simulink model "vbyfcontrolim_trials"  (R2016a)
settings: Solver=ode4  StartTime=0.0  StopTime=20  FixedStep=Ts  RelTol=1e-3
values from neighbouring files (symbols this model uses):
  Cdc = 100e-6    (= 0.0001)    [control_simulation_parameters.m]    (also in pmsm_vbyf_sim_parameters.m = 1.5e-05; vbyfcontrolim_sim.m)
  deltad = delta*180/pi    [control_simulation_parameters.m]    (also in pmsm_vbyf_sim_parameters.m)
  Ef = 155    [control_simulation_parameters.m]    (also in pmsm_vbyf_sim_parameters.m = 80)
  fout = 50    [control_simulation_parameters.m]    (also in pmsm_vbyf_sim_parameters.m = 100; vbyfcontrolim_sim.m)
  frated = 50    [vbyfcontrolim_sim.m]
  Ls = 13.8e-3    (= 0.0138)    [control_simulation_parameters.m]
  ma = Vt*sqrt(3)/(Vdcm*0.612)    [control_simulation_parameters.m]    (also in pmsm_vbyf_sim_parameters.m; vbyfcontrolim_sim.m = 0.9)
  phase = [0 90 0 90]    [control_simulation_parameters.m]    (also in pmsm_vbyf_sim_parameters.m = [0])
  Rin = 10    [control_simulation_parameters.m]    (also in pmsm_vbyf_sim_parameters.m = 1; vbyfcontrolim_sim.m = 1e-06)
  Ripth = 0.08    [control_simulation_parameters.m]    (also in pmsm_vbyf_sim_parameters.m; vbyfcontrolim_sim.m)
  Rs = 1e-3    (= 0.001)    [control_simulation_parameters.m]
  Tload = 30    [pmsm_vbyf_sim_parameters.m]    (also in vbyfcontrolim_sim.m = 10)
  Ts = 100e-9    (= 1e-07)    [control_simulation_parameters.m]    (also in pmsm_vbyf_sim_parameters.m = 1e-06; vbyfcontrolim_sim.m = 1e-06)
  VbyfFreqSteps = 2    [vbyfcontrolim_sim.m]
  VbyfStepTime = 0.2    [vbyfcontrolim_sim.m]
  Vdc = 300    [control_simulation_parameters.m]    (also in pmsm_vbyf_sim_parameters.m = 270; vbyfcontrolim_sim.m = 750)
  Vin = Vdc + Rin*(Pout/Vdc)    (= 366.666666667)    [control_simulation_parameters.m]    (also in pmsm_vbyf_sim_parameters.m = 276.981317008; vbyfcontrolim_sim.m = 750)
  wout = 2*pi*fout    (= 314.159265359)    [control_simulation_parameters.m]    (also in pmsm_vbyf_sim_parameters.m = 628.318530718; vbyfcontrolim_sim.m)
undefined symbols (not defined in the file or in its folder): Lload, Rload
libraries: powerlib x25, powerlib_meascontrol x13, simulink x4, dspsigops x4
settings Model: SimulationMode=accelerator  Creator=ugurm  LastModifiedBy=admin
settings DataIOCC: LimitDataPoints=on  SaveFormat=Array
settings DebuggingCC: UnderspecifiedInitializationDetection=Classic  MergeDetectMultiDrivingBlocksExec=none  SolverPrmCheckMsg=warning  StateNameClashWarn=warning
settings HardwareCC: ProdBitPerPointer=32  ProdLargestAtomicFloat=None  ProdIntDivRoundTo=Undefined  ProdEndianess=Unspecified  ProdWordSize=32  ProdHWDeviceType=32-bit Generic
settings ModelReferenceCC: PropagateSignalLabelsOutOfModel=off
settings SimscapeCC: SimscapeNormalizeSystem=off

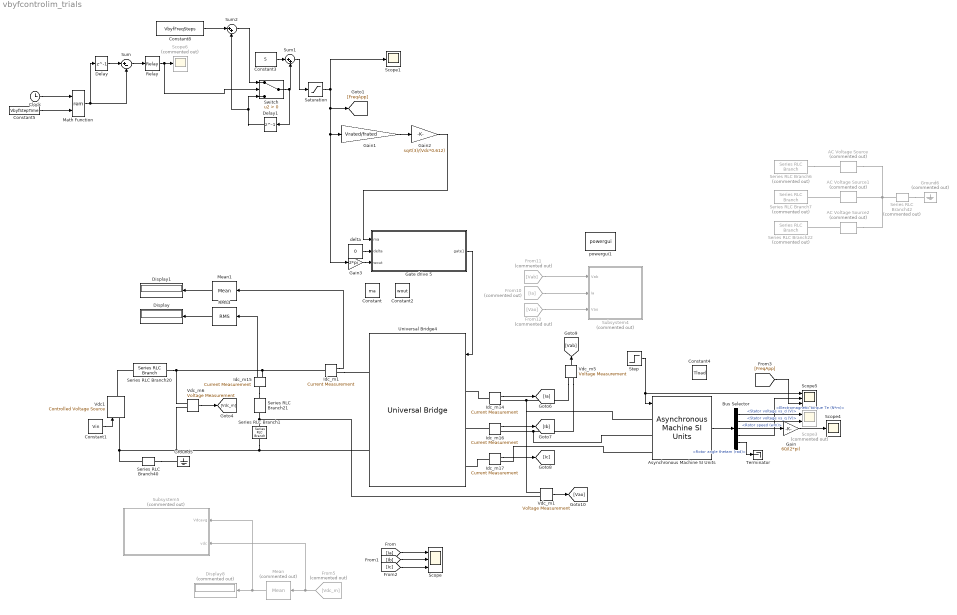
== system vbyfcontrolim_trials ==
  AC Voltage Source : powerlib/Electrical Sources/AC Voltage Source  Commented=on  Amplitude=Ef*sqrt(2)  Phase=0  Frequency=fout  SampleTime=0  Measurements=None  BusType=swing  Pref=10e3  Qref=0  Qmin=-inf  Qmax=+inf
  AC Voltage Source1 : powerlib/Electrical Sources/AC Voltage Source  Commented=on  Amplitude=Ef*sqrt(2)  Phase=-120  Frequency=fout  SampleTime=0  Measurements=None  BusType=swing  Pref=10e3  Qref=0  Qmin=-inf  Qmax=+inf
  AC Voltage Source2 : powerlib/Electrical Sources/AC Voltage Source  Commented=on  Amplitude=Ef*sqrt(2)  Phase=-240  Frequency=fout  SampleTime=0  Measurements=None  BusType=swing  Pref=10e3  Qref=0  Qmin=-inf  Qmax=+inf
  Asynchronous Machine SI Units : powerlib/Machines/Asynchronous Machine SI Units  RotorType=Squirrel-cage  PresetModel=No  MechanicalLoad=Torque Tm  ShowDetailedParameters=on  ReferenceFrame=Synchronous  Units=SI  MeasurementBus=off  NominalParameters=[4000 400 50]  Stator=[1.405 0.005839]  Rotor=[1.395 0.005839]  Cage1=[0.4155 0.002066]  Cage2=[0.4168 0.0003495]  Lm=0.1722  Mechanical=[0.0131 0.002985 2]  PolePairs=2  InitialConditions=[0 0 0 0 0 0 0 0]  SimulateSaturation=off  Saturation=[14.03593122, 27.81365428, 53.79336849, 72.68890987, 97.98006896, 148.6815601, 215.7428561, 302.9841135, 428.7778367 ; 230, 322, 414, 460, 506, 552, 598, 644, 690]  LoadFlowParameters=1492000  TsPowergui=0  TsBlock=-1  IterativeModel=Trapezoidal non iterative  IterativeDiscreteModel=Trapezoidal non iterative  Pmec=1.492e+006
  Bus Selector : BusSelector  OutputSignals=Stator measurements.Stator voltage vs_d (V),Stator measurements.Stator voltage vs_q (V),Mechanical.Rotor speed (wm),Mechanical.Electromagnetic torque Te (N*m),Mechanical.Rotor angle thetam (rad)
  Clock : Clock
  Constant : Constant  Value=ma
  Constant1 : Constant  Value=Vin
  Constant2 : Constant  Value=wout
  Constant3 : Constant  Value=5
  Constant4 : Constant  Value=Tload
  Constant5 : Constant  Value=VbyfStepTime
  Constant8 : Constant  Value=VbyfFreqSteps
  Delay : Delay  DelayLength=1
  Delay1 : Delay  DelayLength=1
  Display : Display
  Display1 : Display
  Display8 : Display  Commented=on
  From10 : From  Commented=on  GotoTag=Ia
  From11 : From  Commented=on  GotoTag=Vab
  From12 : From  Commented=on  GotoTag=Vao
  From5 : From  Commented=on  GotoTag=Vdc_m
  Gain : Gain  Gain=60/(2*pi)
  Gain1 : Gain  Gain=Vrated/frated
  Gain2 : Gain  Gain=sqrt(3)/(Vdc*0.612)
  Gain3 : Gain  Gain=2*pi
  Gate drive 5 : Subsystem
  Ground5 : powerlib/Elements/Ground  LConnTagsString=a
  Ground6 : powerlib/Elements/Ground  Commented=on  LConnTagsString=a
  Idc_m{1,14..17} (5 alike) : powerlib/Measurements/Current Measurement  PhasorSimulation=off  OutputType=Complex  PSBequivalent=0
  Math Function : Math  Operator=rem  SaturateOnIntegerOverflow=on
  Mean : powerlib_meascontrol/Measurements/Mean  Commented=on  Freq=fout  Vinit=0  Ts=0
  Mean1 : powerlib_meascontrol/Measurements/Mean  Freq=fout  Vinit=0  Ts=0
  RMS3 : powerlib_meascontrol/Measurements/RMS  TrueRMS=on  Freq=fout  RMSInit=0  Ts=0
  Relay : Relay
  Saturation : Saturate  UpperLimit=frated  LowerLimit=0
  Scope : Scope  NumInputPorts=3
  Scope1 : Scope
  Scope3 : Scope  Commented=on  NumInputPorts=2
  Scope4 : Scope
  Scope5 : Scope  NumInputPorts=3
  Scope6 : Scope  Commented=on
  Series RLC Branch1 : powerlib/Elements/Series RLC Branch  LConnTagsString=__new0  RConnTagsString=__new0  BranchType=C  Resistance=Rload  Inductance=Lload  SetiL0=off  InitialCurrent=0  Capacitance=Cdc*2  Setx0=off  InitialVoltage=0  Measurements=None
  Series RLC Branch20 : powerlib/Elements/Series RLC Branch  LConnTagsString=__new0  RConnTagsString=__new0  BranchType=R  Resistance=Rin  Inductance=Lload  SetiL0=off  InitialCurrent=0  Capacitance=1e-6  Setx0=off  InitialVoltage=0  Measurements=None
  Series RLC Branch21 : powerlib/Elements/Series RLC Branch  LConnTagsString=__new0  RConnTagsString=__new0  BranchType=C  Resistance=Rload  Inductance=Lload  SetiL0=off  InitialCurrent=0  Capacitance=Cdc*2  Setx0=off  InitialVoltage=0  Measurements=None
  Series RLC Branch22 : powerlib/Elements/Series RLC Branch  Commented=on  LConnTagsString=__new0  RConnTagsString=__new0  BranchType=RL  Resistance=Rs  Inductance=Ls  SetiL0=off  InitialCurrent=0  Capacitance=1e-6  Setx0=off  InitialVoltage=0  Measurements=None
  Series RLC Branch40 : powerlib/Elements/Series RLC Branch  LConnTagsString=__new0  RConnTagsString=__new0  BranchType=R  Resistance=1e12  Inductance=Lload  SetiL0=off  InitialCurrent=0  Capacitance=1e-6  Setx0=off  InitialVoltage=0  Measurements=None
  Series RLC Branch42 : powerlib/Elements/Series RLC Branch  Commented=on  LConnTagsString=__new0  RConnTagsString=__new0  BranchType=R  Resistance=1e12  Inductance=Lload  SetiL0=off  InitialCurrent=0  Capacitance=1e-6  Setx0=off  InitialVoltage=0  Measurements=None
  Series RLC Branch6 : powerlib/Elements/Series RLC Branch  Commented=on  LConnTagsString=__new0  RConnTagsString=__new0  BranchType=RL  Resistance=Rs  Inductance=Ls  SetiL0=off  InitialCurrent=0  Capacitance=1e-6  Setx0=off  InitialVoltage=0  Measurements=None
  Series RLC Branch7 : powerlib/Elements/Series RLC Branch  Commented=on  LConnTagsString=__new0  RConnTagsString=__new0  BranchType=RL  Resistance=Rs  Inductance=Ls  SetiL0=off  InitialCurrent=0  Capacitance=1e-6  Setx0=off  InitialVoltage=0  Measurements=None
  Step : Step  Time=2  After=Tload  SampleTime=0
  Subsystem4 : Subsystem  Commented=on
  Subsystem5 : Subsystem  Commented=on
  Sum : Sum  Inputs=|+-
  Sum1 : Sum  Inputs=|++
  Sum2 : Sum  Inputs=|++
  Switch : Switch  Criteria=u2 > Threshold
  Terminator : Terminator
  Universal Bridge4 : powerlib/Power Electronics/Universal Bridge  Arms=3  SnubberResistance=1e5  SnubberCapacitance=inf  Device=IGBT / Diodes  Ron=1e-6  Lon=0  ForwardVoltages="[  0  0  ]"  ForwardVoltage=0  GTOparameters=[ 10e-6 , 20e-6 ]  IGBTparameters=[0,0]  Measurements=None  Measurements_2=None  converterType=Rectifier
  Vdc1 : powerlib/Electrical Sources/Controlled Voltage Source  Initialize=off  Source_Type=DC  Amplitude=200  Phase=0  Frequency=0  Measurements=None
  Vdc_m1 : powerlib/Measurements/Voltage Measurement  PhasorSimulation=off  OutputType=Complex  PSBequivalent=0
  Vdc_m5 : powerlib/Measurements/Voltage Measurement  PhasorSimulation=off  OutputType=Complex  PSBequivalent=0
  Vdc_m6 : powerlib/Measurements/Voltage Measurement  PhasorSimulation=off  OutputType=Complex  PSBequivalent=0
  delta : Constant  Value=0
  powergui1 : powerlib/powergui  Priority=1  SimulationMode=Discrete  SampleTime=Ts  frequency=60  Iterations=50  frequencyindice=0  Pbase=100e6  ErrMax=1e-4  UnitsV=kV  UnitsW=MW  buscounter=0  FunctionMessages=off  echomessages=off  EnableUseOfTLC=off  CurrentSourceSwitches=off  DisableSnubberDevices=off  DisableRonSwitches=off  DisableVfSwitches=off  DisplayEquations=off  AutomaticDiscreteSolvers=off  SolverType=Tustin  Interpol=off  ExternalGateDelay=off  methode=off  Ts=0  x0status=blocks  SPID=off  SwTol=0  HookPort=off  NonlinearTolerance=0  nMaxIteration=15  ContinueOnMaxIteration=off  RestoreLinks=warning  ResistiveCurrentMeasurement=off  Frange=[0:2:500]  Ylog=off  Xlog=on  ShowGrid=off  save=off  variable=ZData  structure=Vdc  ZoomFFT=off  StartTime=0.04  cycles=5  DisplayStyle=5  fundamental=50  FreqAxis=off  MaxFrequency=30000  frequencyindicesteady=1  RmsSteady=1  display=off
  wires:
  Gate drive 5/1(gate1) -> Universal Bridge4/1
  Constant1/1 -> Vdc1/1
  Idc_m15/1 -> RMS3/1
  Vdc_m6/1 -> [Vdc_m]
  RMS3/1 -> Display/1
  Mean/1 -> Subsystem5/1(Vdcavg), Display8/1
  Idc_m1/1 -> Mean1/1
  Mean1/1 -> Display1/1
  Idc_m14/1 -> [Ia]
  From5/1 -> Subsystem5/2(vdc), Mean/1
  From10/1 -> Subsystem4/2(Ia)
  Idc_m16/1 -> [Ib]
  Idc_m17/1 -> [Ic]
  From11/1 -> Subsystem4/1(Vab)
  From12/1 -> Subsystem4/3(Vao)
  Vdc_m5/1 -> [Vab]
  Vdc_m1/1 -> [Vao]
  [Ia] -> Scope/1
  [Ic] -> Scope/3
  [Ib] -> Scope/2
  delta/1 -> Gate drive 5/2(delta)
  Asynchronous Machine SI Units/1 -> Bus Selector/1
  Bus Selector/1 -> Scope3/1  "<Stator voltage vs_d (V)>"
  Bus Selector/2 -> Scope3/2  "<Stator voltage vs_q (V)>"
  Bus Selector/3 -> Gain/1  "<Rotor speed (wm)>"
  Bus Selector/4 -> Scope5/2  "<Electromagnetic torque Te (N*m)>"
  Bus Selector/5 -> Terminator/1  "<Rotor angle thetam (rad)>"
  Gain/1 -> Scope4/1
  Clock/1 -> Math Function/1
  Constant5/1 -> Math Function/2
  Math Function/1 -> Sum/2, Delay/1
  Delay/1 -> Sum/1
  Sum/1 -> Relay/1
  Relay/1 -> Switch/2, Scope6/1
  Sum2/1 -> Switch/1
  Constant8/1 -> Sum2/1
  Delay1/1 -> Switch/3, Sum2/2
  Switch/1 -> Sum1/2, Delay1/1
  Gain1/1 -> Gain2/1
  Gain2/1 -> Gate drive 5/1(ma)
  Gain3/1 -> Gate drive 5/3(wout)
  Saturation/1 -> [FreqApp], Gain3/1, Gain1/1, Scope1/1
  Step/1 -> Scope5/1, Asynchronous Machine SI Units/1
  [FreqApp] -> Scope5/3
  Constant3/1 -> Sum1/1
  Sum1/1 -> Saturation/1
  connections:
  Vdc_m5/LConn1 -- Asynchronous Machine SI Units/LConn1 -- Vdc_m1/LConn1 -- Idc_m14/RConn1
  Universal Bridge4/RConn2 -- Vdc_m6/LConn2 -- Vdc1/LConn1 -- Series RLC Branch40/LConn1 -- Series RLC Branch1/RConn1
  Series RLC Branch42/RConn1 -- Ground6/LConn1
  Series RLC Branch40/RConn1 -- Ground5/LConn1
  Idc_m14/LConn1 -- Universal Bridge4/LConn1
  Idc_m15/LConn1 -- Series RLC Branch21/LConn1
  Vdc1/RConn1 -- Series RLC Branch20/LConn1
  Series RLC Branch6/RConn1 -- AC Voltage Source/RConn1
  AC Voltage Source1/RConn1 -- Series RLC Branch7/RConn1
  AC Voltage Source2/RConn1 -- Series RLC Branch22/RConn1
  Series RLC Branch42/LConn1 -- AC Voltage Source/LConn1 -- AC Voltage Source2/LConn1 -- AC Voltage Source1/LConn1
  Idc_m16/LConn1 -- Universal Bridge4/LConn2
  Idc_m17/LConn1 -- Universal Bridge4/LConn3
  Vdc_m5/LConn2 -- Asynchronous Machine SI Units/LConn2 -- Idc_m16/RConn1
  Idc_m1/RConn1 -- Universal Bridge4/RConn1
  Idc_m1/LConn1 -- Series RLC Branch20/RConn1 -- Vdc_m6/LConn1 -- Idc_m15/RConn1
  Series RLC Branch1/LConn1 -- Vdc_m1/LConn2 -- Series RLC Branch21/RConn1
  Asynchronous Machine SI Units/LConn3 -- Idc_m17/RConn1

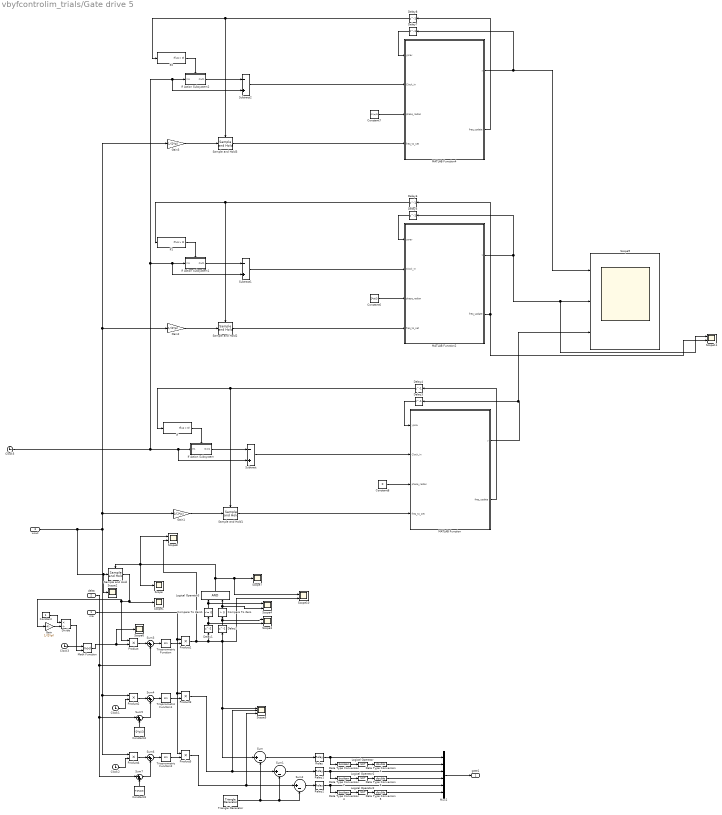
== system vbyfcontrolim_trials/Gate drive 5 ==
  ma : Inport
  delta : Inport  Port=2
  wout : Inport  Port=3
  Clock{1..3,5} (4 alike) : Clock
  Compare To Zero : simulink/Logic and Bit Operations/Compare To Zero  relop=>  OutDataTypeStr=boolean
  Compare To Zero1 : simulink/Logic and Bit Operations/Compare To Zero  relop=<=  OutDataTypeStr=boolean
  Constant : Constant
  Constant3 : Constant  Value=+2*pi/3
  Constant4 : Constant  Value=-2*pi/3
  Constant6 : Constant  Value=2*pi/3
  Constant7 : Constant  Value=-2*pi/3
  Constant8 : Constant  Value=0
  Data Type Conversion : DataTypeConversion  OutDataTypeStr=boolean
  Data Type Conversion1 : DataTypeConversion  OutDataTypeStr=double
  Data Type Conversion2 : DataTypeConversion  OutDataTypeStr=boolean
  Data Type Conversion3 : DataTypeConversion  OutDataTypeStr=double
  Data Type Conversion4 : DataTypeConversion  OutDataTypeStr=boolean
  Data Type Conversion5 : DataTypeConversion  OutDataTypeStr=double
  Delay1 : Delay
  Delay{2..8} (7 alike) : Delay  DelayLength=1
  Divide : Product  Inputs=*/
  Gain{,1..3} (4 alike) : Gain  Gain=1/(2*pi)
  If : If  ShowElse=off
  If Action Subsystem : Subsystem  TreatAsAtomicUnit=on
  If Action Subsystem1 : Subsystem  TreatAsAtomicUnit=on
  If Action Subsystem2 : Subsystem  TreatAsAtomicUnit=on
  If1 : If  ShowElse=off
  If2 : If  ShowElse=off
  Logical Operator : Logic  Operator=NOT  AllPortsSameDT=off  OutDataTypeStr=boolean
  Logical Operator1 : Logic  Operator=NOT  AllPortsSameDT=off  OutDataTypeStr=boolean
  Logical Operator2 : Logic  Operator=NOT  AllPortsSameDT=off  OutDataTypeStr=boolean
  Logical Operator3 : Logic  AllPortsSameDT=off  OutDataTypeStr=boolean
  MATLAB Function : MATLAB Function  TreatAsAtomicUnit=on
  MATLAB Function2 : MATLAB Function  TreatAsAtomicUnit=on
  MATLAB Function4 : MATLAB Function  TreatAsAtomicUnit=on
  Math Function : Math  Operator=mod  SaturateOnIntegerOverflow=on
  Mux2 : Mux  Inputs=6
  Product{,1..5} (6 alike) : Product
  Relay : Relay
  Relay1 : Relay
  Relay2 : Relay
  Sample and Hold{,1..3} (4 alike) : dspsigops/Sample and Hold  trig=Rising edge  initCond=5*2*pi  latchinput=off
  Scope{,1..2,6..7} (5 alike) : Scope
  Scope{3..4,8,10..11} (5 alike) : Scope  NumInputPorts=2
  Scope5 : Scope  NumInputPorts=3
  Scope9 : Scope  NumInputPorts=3
  Subtract : Sum  Inputs=-+
  Subtract1 : Sum  Inputs=-+
  Subtract2 : Sum  Inputs=-+
  Sum : Sum  Inputs=|+-
  Sum1 : Sum  Inputs=|+-
  Sum2 : Sum  Inputs=|+-
  Sum{3..7} (5 alike) : Sum  Inputs=|++
  Triangle Generator : powerlib_meascontrol/Pulse & Signal Generators/Triangle Generator  Freq=fsw  Phase=phase(1)  Ts=Ts
  Trigonometric Function : Trigonometry
  Trigonometric Function1 : Trigonometry
  Trigonometric Function2 : Trigonometry
  gate1 : Outport
  wires:
  Triangle Generator/1 -> Sum1/2, Sum2/2, Sum/2
  Product3/1 -> Scope5/2, Sum1/1
  Product5/1 -> Scope5/3, Sum2/1
  Sum/1 -> Relay/1
  Sum1/1 -> Relay1/1
  Sum2/1 -> Relay2/1
  Data Type Conversion/1 -> Logical Operator/1
  Relay/1 -> Data Type Conversion/1, Mux2/1
  Logical Operator/1 -> Data Type Conversion1/1
  Data Type Conversion1/1 -> Mux2/2
  Data Type Conversion2/1 -> Logical Operator1/1
  Relay1/1 -> Data Type Conversion2/1, Mux2/3
  Logical Operator1/1 -> Data Type Conversion3/1
  Data Type Conversion3/1 -> Mux2/4
  Data Type Conversion4/1 -> Logical Operator2/1
  Relay2/1 -> Data Type Conversion4/1, Mux2/5
  Logical Operator2/1 -> Data Type Conversion5/1
  Data Type Conversion5/1 -> Mux2/6
  Mux2/1 -> gate1/1
  Trigonometric Function/1 -> Product1/2
  Sum3/1 -> Trigonometric Function/1
  Product/1 -> Sum3/1
  Clock1/1 -> Product2/2
  Trigonometric Function1/1 -> Product3/2
  Sum4/1 -> Trigonometric Function1/1
  Product2/1 -> Sum4/1
  Sum5/1 -> Sum4/2
  Constant4/1 -> Sum5/2
  ma/1 -> Product1/1, Product5/1, Product3/1
  delta/1 -> Sum7/1, Sum5/1, Sum3/2
  Clock2/1 -> Product4/2
  Trigonometric Function2/1 -> Product5/2
  Sum6/1 -> Trigonometric Function2/1
  Product4/1 -> Sum6/1
  Sum7/1 -> Sum6/2
  Constant3/1 -> Sum7/2
  Sample and Hold/1 -> Scope1/1, Product/1, Gain/1
  Product1/1 -> Scope8/2, Delay1/1, Scope10/2, Scope5/1, Sum/1, Delay2/1
  Delay1/1 -> Compare To Zero1/1, Scope3/2
  Compare To Zero/1 -> Scope4/2, Logical Operator3/2
  Compare To Zero1/1 -> Scope4/1, Logical Operator3/1
  Delay2/1 -> Scope3/1, Compare To Zero/1
  Gain/1 -> Divide/2
  Constant/1 -> Divide/1
  Divide/1 -> Math Function/2
  Clock3/1 -> Math Function/1
  Math Function/1 -> Scope6/1, Product/2
  Logical Operator3/1 -> Scope10/1, Scope7/1, Scope8/1, Scope/1, Sample and Hold/Trigger
  MATLAB Function/1(y) -> Scope9/3, Delay3/1
  Delay3/1 -> MATLAB Function/1(yprev)
  MATLAB Function/2(freq_update) -> Delay4/1
  Gain1/1 -> Sample and Hold1/1
  Sample and Hold1/1 -> MATLAB Function/4(freq_to_set)
  Delay4/1 -> Sample and Hold1/Trigger, If/1
  If Action Subsystem/1(Out1) -> Subtract/1
  If/1 -> If Action Subsystem/Action
  Subtract/1 -> MATLAB Function/2(Clock_In)
  Subtract1/1 -> MATLAB Function2/2(Clock_In)
  If1/1 -> If Action Subsystem1/Action
  If Action Subsystem1/1(Out1) -> Subtract1/1
  Delay6/1 -> If1/1, Sample and Hold2/Trigger
  Sample and Hold2/1 -> MATLAB Function2/4(freq_to_set)
  Gain2/1 -> Sample and Hold2/1
  MATLAB Function2/2(freq_update) -> Scope11/2, Delay6/1
  Delay5/1 -> MATLAB Function2/1(yprev)
  MATLAB Function2/1(y) -> Scope11/1, Scope9/2, Delay5/1
  MATLAB Function4/1(y) -> Scope9/1, Delay7/1
  Delay7/1 -> MATLAB Function4/1(yprev)
  MATLAB Function4/2(freq_update) -> Delay8/1
  If Action Subsystem2/1(Out1) -> Subtract2/1
  Sample and Hold3/1 -> MATLAB Function4/4(freq_to_set)
  Gain3/1 -> Sample and Hold3/1
  Delay8/1 -> If2/1, Sample and Hold3/Trigger
  Subtract2/1 -> MATLAB Function4/2(Clock_In)
  Clock5/1 -> Subtract/2, If Action Subsystem/1(In1), If Action Subsystem1/1(In1), Subtract1/2, If Action Subsystem2/1(In1), Subtract2/2
  If2/1 -> If Action Subsystem2/Action
  wout/1 -> Scope2/1, Sample and Hold/1, Product4/1, Product2/1, Gain3/1, Gain2/1, Gain1/1
  Constant6/1 -> MATLAB Function2/3(phase_radian)
  Constant7/1 -> MATLAB Function4/3(phase_radian)
  Constant8/1 -> MATLAB Function/3(phase_radian)

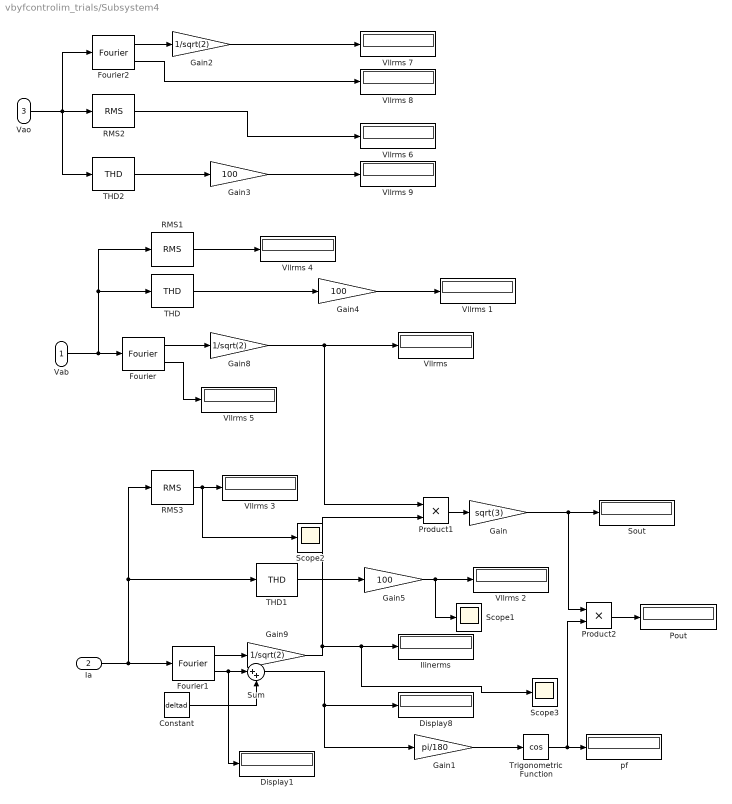
== system vbyfcontrolim_trials/Subsystem4 ==
  Vab : Inport
  Ia : Inport  Port=2
  Vao : Inport  Port=3
  Constant : Constant  Value=deltad
  Display1 : Display
  Display8 : Display
  Fourier : powerlib_meascontrol/Measurements/Fourier  Freq=fout  n=1  InInit=[0, 0]  Ts=Ts
  Fourier1 : powerlib_meascontrol/Measurements/Fourier  Freq=fout  n=1  InInit=[0, 0]  Ts=Ts
  Fourier2 : powerlib_meascontrol/Measurements/Fourier  Freq=fout  n=1  InInit=[0, 0]  Ts=Ts
  Gain : Gain  Gain=sqrt(3)
  Gain1 : Gain  Gain=pi/180
  Gain2 : Gain  Gain=1/sqrt(2)
  Gain3 : Gain  Gain=100
  Gain4 : Gain  Gain=100
  Gain5 : Gain  Gain=100
  Gain8 : Gain  Gain=1/sqrt(2)
  Gain9 : Gain  Gain=1/sqrt(2)
  "Ilinerms " : Display
  Pout : Display
  Product1 : Product
  Product2 : Product
  RMS1 : powerlib_meascontrol/Measurements/RMS  TrueRMS=on  Freq=fout  RMSInit=0  Ts=0
  RMS2 : powerlib_meascontrol/Measurements/RMS  TrueRMS=on  Freq=fout  RMSInit=0  Ts=0
  RMS3 : powerlib_meascontrol/Measurements/RMS  TrueRMS=on  Freq=fout  RMSInit=0  Ts=0
  Scope1 : Scope
  Scope2 : Scope
  Scope3 : Scope
  Sout : Display
      settings: Format=short_e
  Sum : Sum  Inputs=|++
  THD : powerlib_meascontrol/Measurements/THD  Freq=fout  Ts=0
  THD1 : powerlib_meascontrol/Measurements/THD  Freq=fout  Ts=0
  THD2 : powerlib_meascontrol/Measurements/THD  Freq=fout  Ts=0
  Trigonometric Function : Trigonometry  Operator=cos
  Vllrms {,1..9} (10 alike) : Display
  pf : Display
  wires:
  Gain8/1 -> Product1/1, "Vllrms "/1
  Gain9/1 -> Scope3/1, "Ilinerms "/1, Product1/2
  Ia/1 -> RMS3/1, THD1/1, Fourier1/1
  Fourier1/1 -> Gain9/1
  Vab/1 -> RMS1/1, THD/1, Fourier/1
  Fourier/1 -> Gain8/1
  Product1/1 -> Gain/1
  Gain/1 -> Product2/1, Sout/1
  Sum/1 -> Gain1/1, Display8/1
  Trigonometric Function/1 -> Product2/2, pf/1
  Gain1/1 -> Trigonometric Function/1
  Product2/1 -> Pout/1
  Fourier/2 -> Vllrms 5/1
  THD/1 -> Gain4/1
  THD1/1 -> Gain5/1
  Constant/1 -> Sum/2
  RMS3/1 -> Scope2/1, Vllrms 3/1
  RMS1/1 -> Vllrms 4/1
  Fourier1/2 -> Display1/1, Sum/1
  Vao/1 -> THD2/1, Fourier2/1, RMS2/1
  RMS2/1 -> Vllrms 6/1
  Fourier2/1 -> Gain2/1
  Fourier2/2 -> Vllrms 8/1
  Gain2/1 -> Vllrms 7/1
  THD2/1 -> Gain3/1
  Gain3/1 -> Vllrms 9/1
  Gain4/1 -> Vllrms 1/1
  Gain5/1 -> Scope1/1, Vllrms 2/1

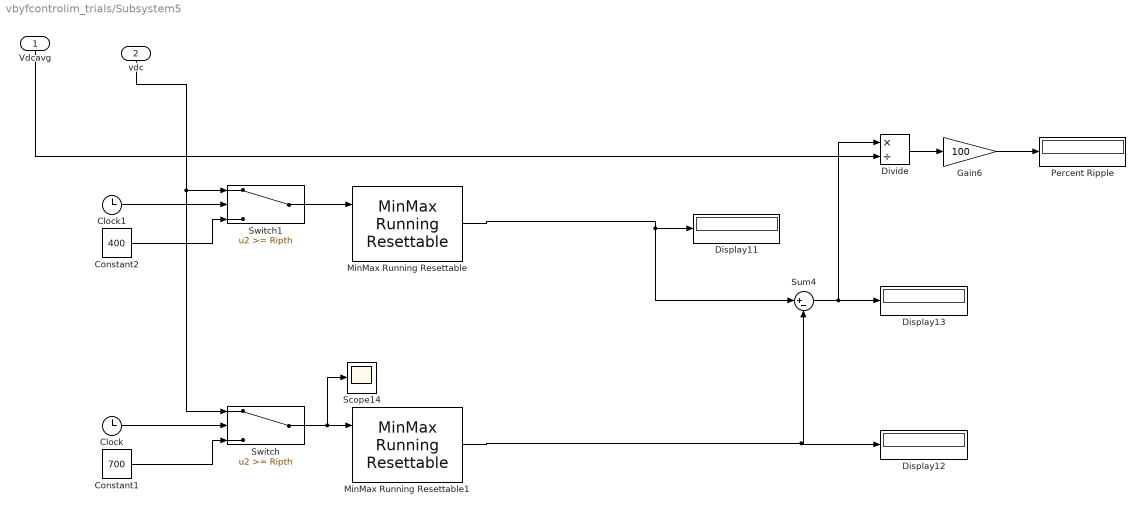
== system vbyfcontrolim_trials/Subsystem5 ==
  Vdcavg : Inport
  vdc : Inport  Port=2
  Clock : Clock
  Clock1 : Clock
  Constant1 : Constant  Value=700  SampleTime=Ts
  Constant2 : Constant  Value=400  SampleTime=Ts
  Display11 : Display
  Display12 : Display
  Display13 : Display
  Divide : Product  Inputs=*/
  Gain6 : Gain  Gain=100
  MinMax Running Resettable : simulink/Math Operations/MinMax Running Resettable  Function=max  vinit=0.0
  MinMax Running Resettable1 : simulink/Math Operations/MinMax Running Resettable  Function=min  vinit=700
  Percent Ripple : Display
  Scope14 : Scope
  Sum4 : Sum  Inputs=|+-
  Switch : Switch  Threshold=Ripth
  Switch1 : Switch  Threshold=Ripth
  wires:
  MinMax Running Resettable/1 -> Display11/1, Sum4/1
  Clock/1 -> Switch/2
  Gain6/1 -> Percent Ripple/1
  Constant1/1 -> Switch/3
  MinMax Running Resettable1/1 -> Display12/1, Sum4/2
  Switch/1 -> Scope14/1, MinMax Running Resettable1/1
  Sum4/1 -> Divide/1, Display13/1
  Divide/1 -> Gain6/1
  Vdcavg/1 -> Divide/2
  vdc/1 -> Switch1/1, Switch/1
  Switch1/1 -> MinMax Running Resettable/1
  Clock1/1 -> Switch1/2
  Constant2/1 -> Switch1/3

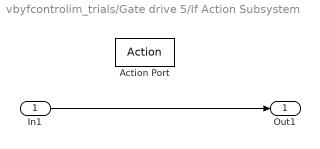
== system vbyfcontrolim_trials/Gate drive 5/If Action Subsystem ==
  In1 : Inport
  Action Port : ActionPort
  Out1 : Outport
  wires:
  In1/1 -> Out1/1

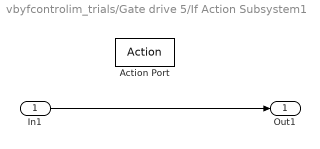
== system vbyfcontrolim_trials/Gate drive 5/If Action Subsystem1 ==
  In1 : Inport
  Action Port : ActionPort
  Out1 : Outport
  wires:
  In1/1 -> Out1/1

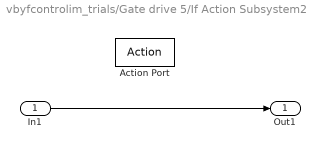
== system vbyfcontrolim_trials/Gate drive 5/If Action Subsystem2 ==
  In1 : Inport
  Action Port : ActionPort
  Out1 : Outport
  wires:
  In1/1 -> Out1/1

== matlab function vbyfcontrolim_trials/Gate drive 5/MATLAB Function ==
  data: yprev input; y output; Clock_In input; phase_radian input; freq_to_set input; freq_update output
function [y,freq_update]  = fcn(yprev,Clock_In,phase_radian,freq_to_set)
y = sin(2*pi*freq_to_set*Clock_In+phase_radian);
if((yprev<0)&&(y>=0))
    freq_update = 1;
    
else
    freq_update = 0;
    
end

== matlab function vbyfcontrolim_trials/Gate drive 5/MATLAB Function2 ==
  data: yprev input; y output; Clock_In input; phase_radian input; freq_to_set input; freq_update output
function [y,freq_update]  = fcn(yprev,Clock_In,phase_radian,freq_to_set)
y = sin(2*pi*freq_to_set*Clock_In+phase_radian);
if((yprev>sin(phase_radian))&&(y<=sin(phase_radian)))
    freq_update = 1;
    
else
    freq_update = 0;
    
end

== matlab function vbyfcontrolim_trials/Gate drive 5/MATLAB Function4 ==
  data: yprev input; y output; Clock_In input; phase_radian input; freq_to_set input; freq_update output
function [y,freq_update]  = fcn(yprev,Clock_In,phase_radian,freq_to_set)
y = sin(2*pi*freq_to_set*Clock_In+phase_radian);
if((yprev>sin(phase_radian))&&(y<=sin(phase_radian)))
    freq_update = 1;
    
else
    freq_update = 0;
    
end
